simulink model "test_chan_sel"  (Simulink 7.8)
settings: Solver=ode45  StartTime=0.0  StopTime=512  RelTol=1e-3
libraries: xbsIndex_r4 x128, casper_library_misc x14, xps_library x9, simulink x4
settings Model: Creator=dprice  LastModifiedBy=dprice

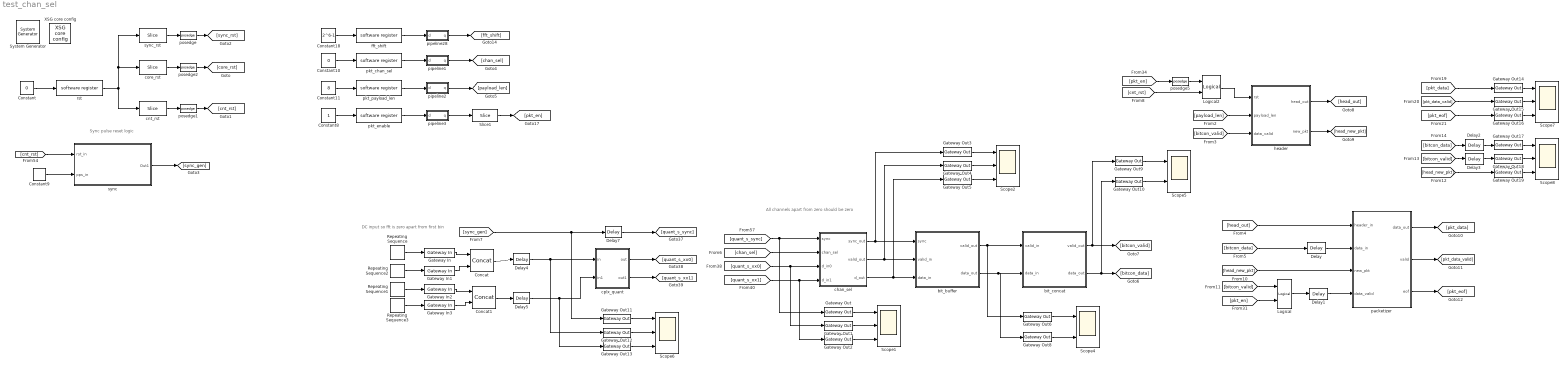
== system test_chan_sel ==
  note: Sync pulse reset logic
  note: DC input so fft is zero apart from first bin
  note: All channels apart from zero should be zero
  " System Generator" : xbsIndex_r4/ System Generator  Tag=genX  xilinxfamily=virtex5  part=xc5vsx95t  speed=-1  package=ff1136  synthesis_tool=XST  clock_wrapper=Clock Enables  directory=./zoom_adc_single_pol/sysgen  proj_type=Project Navigator  Synth_file=XST Defaults  Impl_file=ISE Defaults  testbench=off  simulink_period=1  sysclk_period=5  dcm_input_clock_period=100  incr_netlist=off  trim_vbits=Everywhere in SubSystem  dbl_ovrd=According to Block Masks  core_generation=According to Block Masks  run_coregen=off  deprecated_control=off  eval_field=0  block_type=sysgen
  Concat : xbsIndex_r4/Concat  num_inputs=2  dbl_ovrd=off  block_type=concat
  Concat1 : xbsIndex_r4/Concat  num_inputs=2  dbl_ovrd=off  block_type=concat
  Constant : Constant  Value=0
  Constant10 : Constant  Value=0
  Constant11 : Constant  Value=8
  Constant18 : Constant  Value=2^6-1
  Constant8 : Constant
  Constant9 : xbsIndex_r4/Constant  const=0  gui_display_data_type=Boolean  arith_type=Boolean  n_bits=8  bin_pt=6  preci_type=Single  exp_width=8  frac_width=24  explicit_period=on  period=1  equ=P=C  opselect=C  inp2=PCIN>>17  opr=+  inp1=P  carry=CIN  dbl_ovrd=off  block_type=constant
  Delay{,1..5} (6 alike) : xbsIndex_r4/Delay  rst=off  infoeditControl=Selection of Reset will increase slice count due to use of real FFs and instead of SRLs  en=off  latency=1  dbl_ovrd=off  reg_retiming=off  block_type=delay
  Delay7 : xbsIndex_r4/Delay  rst=off  infoeditControl=Selection of Reset will increase slice count due to use of real FFs and instead of SRLs  en=off  latency=3  dbl_ovrd=off  reg_retiming=off  block_type=delay
  Gateway In{,1..3} (4 alike) : xbsIndex_r4/Gateway In  gui_display_data_type=Fixed-point  arith_type=Unsigned  n_bits=18  bin_pt=0  preci_type=Single  exp_width=8  frac_width=24  quantization="Round  (unbiased: +/- Inf)"  overflow=Saturate  period=1  dbl_ovrd=off  timing_constraint=None  locs_specified=off  LOCs={}  inherit_from_input=off  UseAsADC=off  ADCChannel='1'  hdl_port=on  block_type=gatewayin
      settings: infoedit="Gateway in block.  Converts inputs of type Simulink integer, single, double and fixed point to  Xilinx fixed-point or floating-point data type.<br><br>Hardware notes:  In hardware these blocks become top level input ports."
  Gateway Out{,1..6,8..19} (19 alike) : xbsIndex_r4/Gateway Out  inherit_from_input=off  hdl_port=on  timing_constraint=None  locs_specified=off  LOCs={}  UseAsDAC=off  DACChannel='1'  block_type=gatewayout
      settings: infoedit="Gateway out block.  Converts Xilinx fixed-point or floating-point type inputs into ouputs of type Simulink integer, single, double, or fixed point.<br><br>Hardware notes:  In hardware these blocks become top level output ports or are discarded, depending on how they are configured."
  Logical : xbsIndex_r4/Logical  logical_function=AND  inputs=2  en=off  latency=0  precision=Full  arith_type=Unsigned  n_bits=16  bin_pt=0  align_bp=on  dbl_ovrd=off  block_type=logical
  Logical2 : xbsIndex_r4/Logical  logical_function=OR  inputs=2  en=off  latency=0  precision=Full  arith_type=Unsigned  n_bits=16  bin_pt=0  align_bp=on  dbl_ovrd=off  block_type=logical
  Repeating Sequence : simulink/Sources/Repeating Sequence  rep_seq_t=[1 2 3 4 5 6 7 8 9]  rep_seq_y=[128 0 0 0 0 0 0 0 0]
  Repeating Sequence1 : simulink/Sources/Repeating Sequence  rep_seq_t=[1 2 3 4 5 6 7 8]  rep_seq_y=[0 0 0 0 0 0 0 0]
  Repeating Sequence2 : simulink/Sources/Repeating Sequence  rep_seq_t=[1 2 3 4 5 6 7 8 9]  rep_seq_y=[128 0 0 0 0 0 0 0 0]
  Repeating Sequence3 : simulink/Sources/Repeating Sequence  rep_seq_t=[1 2 3 4 5 6 7 8]  rep_seq_y=[0 0 0 0 0 0 0 0]
  Scope{1..2,6..8} (5 alike) : Scope  NumInputPorts=3
      Scope1 settings: YMin=-5~-5~-5  YMax=5~5~5
      Scope2 settings: YMin=-5~-5~-5  YMax=5~5~5  SaveName=ScopeData6
      Scope6 settings: YMin=-5~-5~-5  YMax=5~5~5  SaveName=ScopeData10
      Scope7 settings: TimeRange=290.1459854014598  YMin=9.44473e+21~0~-1  YMax=3.5e+38~1~1  SaveName=ScopeData11
      Scope8 settings: TimeRange=290.1459854014598  YMin=0~0~0  YMax=1.2e+18~1~1  SaveName=ScopeData12
  Scope4 : Scope  NumInputPorts=2
      settings: YMin=-5~-5  YMax=5~5  SaveName=ScopeData8
  Scope5 : Scope  NumInputPorts=2
      settings: YMin=-5~-5  YMax=5~5  SaveName=ScopeData9
  Slice1 : xbsIndex_r4/Slice  nbits=1  boolean_output=on  mode=Lower Bit Location + Width  bit1=1  base1=MSB of Input  bit0=0  base0=LSB of Input  dbl_ovrd=off  block_type=slice
      settings: block_version=10.1.3
  XSG core config : xps_library/XSG core config  Tag=xps:xsg  hw_sys=ROACH:sx95t  ibob_linux=off  clk_src=adc0_clk  iBOB_clk_src=sys_clk  BEE2_ctrl_clk_src=sys_clk  BEE2_usr_clk_src=sys_clk  ROACH_clk_src=adc0_clk  ROACH2_clk_src=adc0_clk  CORR_clk_src=sys_clk  gpio_clk_io_group=iBOB:sma  gpio_clk_bit_index=0  clk_rate=200  sample_period=1  synthesis_tool=XST  mpc_type=powerpc440_ext
  bit_buffer : Subsystem
  bit_concat : Subsystem
  chan_sel : Subsystem
  cnt_rst : xbsIndex_r4/Slice  nbits=1  boolean_output=on  mode=Lower Bit Location + Width  bit1=0  base1=MSB of Input  bit0=0  base0=LSB of Input  dbl_ovrd=off  block_type=slice
  core_rst : xbsIndex_r4/Slice  nbits=1  boolean_output=on  mode=Lower Bit Location + Width  bit1=0  base1=MSB of Input  bit0=1  base0=LSB of Input  dbl_ovrd=off  block_type=slice
  cplx_quant : Subsystem  AncestorBlock=hipsr_library/quant
  fft_shift : xps_library/software register  Tag=xps:sw_reg  io_dir=From Processor  arith_type=Unsigned  bitwidth=32  bin_pt=0  sample_period=1  gw_name=test_chan_sel_fft_shift_user_data_out
      link override coarse_r01_acc_len_user_data_out: arith_type=Unsigned  n_bits=32  bin_pt=0  period=1
      link override coarse_r02_acc_len_user_data_out: arith_type=Unsigned  n_bits=32  bin_pt=0  period=1
      link override coarse_r03_acc_len_user_data_out: arith_type=Unsigned  n_bits=32  bin_pt=0  period=1
      link override coarse_r04_acc_len_user_data_out: arith_type=Unsigned  n_bits=32  bin_pt=0  period=1
      link override coarse_r06_acc_len_user_data_out: arith_type=Unsigned  n_bits=32  bin_pt=0  period=1
      link override coarse_r07_acc_len_user_data_out: arith_type=Unsigned  n_bits=32  bin_pt=0  period=1
      link override coarse_r08_acc_len_user_data_out: arith_type=Unsigned  n_bits=32  bin_pt=0  period=1
      link override coarse_r09_acc_len_user_data_out: arith_type=Unsigned  n_bits=32  bin_pt=0  period=1
      link override coarse_r10_acc_len_user_data_out: arith_type=Unsigned  n_bits=32  bin_pt=0  period=1
      link override coarse_r12_acc_len_user_data_out: arith_type=Unsigned  n_bits=32  bin_pt=0  period=1
      link override convert: arith_type=Unsigned  n_bits=32  bin_pt=0
      link override qdr_single_r01_acc_len_coarse_user_data_out: arith_type=Unsigned  n_bits=32  bin_pt=0  period=1
      link override qdr_single_r02_acc_len_coarse_user_data_out: arith_type=Unsigned  n_bits=32  bin_pt=0  period=1
      link override qdr_single_r04_acc_len_coarse_user_data_out: arith_type=Unsigned  n_bits=32  bin_pt=0  period=1
      link override r_spec_2048_r102_acc_len_user_data_out: arith_type=Unsigned  n_bits=32  bin_pt=0  period=1
      link override r_spec_2048_r102_nosim_acc_len_user_data_out: arith_type=Unsigned  n_bits=32  bin_pt=0  period=1
      link override r_spec_2048_r103_acc_len_user_data_out: arith_type=Unsigned  n_bits=32  bin_pt=0  period=1
      link override r_spec_2048_r104_acc_len_user_data_out: arith_type=Unsigned  n_bits=32  bin_pt=0  period=1
      link override r_spec_2048_r104_test0_acc_len_user_data_out: arith_type=Unsigned  n_bits=32  bin_pt=0  period=1
      link override r_spec_2048_r104_test_acc_len_user_data_out: arith_type=Unsigned  n_bits=32  bin_pt=0  period=1
      link override r_spec_2048_r105_acc_len_user_data_out: arith_type=Unsigned  n_bits=32  bin_pt=0  period=1
      link override r_spec_test0_acc_len_user_data_out: arith_type=Unsigned  n_bits=32  bin_pt=0  period=1
      link override r_spec_test4_acc_len_user_data_out: arith_type=Unsigned  n_bits=32  bin_pt=0  period=1
      link override roach_spec_acc_len_user_data_out: arith_type=Unsigned  n_bits=32  bin_pt=0  period=1
      link override roach_spec_no10gbe_acc_len_user_data_out: arith_type=Unsigned  n_bits=32  bin_pt=0  period=1
      link override roach_spec_rst_sync_cnt_user_data_out: arith_type=Unsigned  n_bits=32  bin_pt=0  period=1
      link override toast_256ch_16bit_r02_acc_len_user_data_out: arith_type=Unsigned  n_bits=32  bin_pt=0  period=1
      link override toast_256ch_16bit_r04_acc_len_user_data_out: arith_type=Unsigned  n_bits=32  bin_pt=0  period=1
      link override toast_256ch_16bit_r05_acc_len_user_data_out: arith_type=Unsigned  n_bits=32  bin_pt=0  period=1
  header : Subsystem
  packetizer : Subsystem
  pipeline1 : Subsystem  AncestorBlock=casper_library_delays/pipeline  mask(pipeline){latency=1}
      mask help:
      | An explicitly laid-out delay line to avoid mapping to SRL16s
      | for use in pipelining to help achieve timing closure.
      mask init:
      | pipeline_init(gcb,'latency',latency);
      settings: AttributesFormatString=Latency = %<latency>
      mask Display:
      | port_label('input', 1, 'd');
      | port_label('output', 1, 'q');
      | disp(['Z^-', num2str(latency)]);
  pipeline2 : Subsystem  AncestorBlock=casper_library_delays/pipeline  mask(pipeline){latency=1}
      mask help:
      | An explicitly laid-out delay line to avoid mapping to SRL16s
      | for use in pipelining to help achieve timing closure.
      mask init:
      | pipeline_init(gcb,'latency',latency);
      settings: AttributesFormatString=Latency = %<latency>
      mask Display:
      | port_label('input', 1, 'd');
      | port_label('output', 1, 'q');
      | disp(['Z^-', num2str(latency)]);
  pipeline28 : Subsystem  AncestorBlock=casper_library_delays/pipeline  mask(pipeline){latency=1}
      mask help:
      | An explicitly laid-out delay line to avoid mapping to SRL16s
      | for use in pipelining to help achieve timing closure.
      mask init:
      | pipeline_init(gcb,'latency',latency);
      settings: AttributesFormatString=Latency = %<latency>
      mask Display:
      | port_label('input', 1, 'd');
      | port_label('output', 1, 'q');
      | disp(['Z^-', num2str(latency)]);
  pipeline3 : Subsystem  AncestorBlock=casper_library_delays/pipeline  mask(pipeline){latency=1}
      mask help:
      | An explicitly laid-out delay line to avoid mapping to SRL16s
      | for use in pipelining to help achieve timing closure.
      mask init:
      | pipeline_init(gcb,'latency',latency);
      settings: AttributesFormatString=Latency = %<latency>
      mask Display:
      | port_label('input', 1, 'd');
      | port_label('output', 1, 'q');
      | disp(['Z^-', num2str(latency)]);
  pkt_chan_sel : xps_library/software register  Tag=xps:sw_reg  io_dir=From Processor  arith_type=Unsigned  bitwidth=32  bin_pt=0  sample_period=1  gw_name=test_chan_sel_pkt_chan_sel_user_data_out
      link override hipsr_tgbe3_pkt_chan_sel_user_data_out: arith_type=Unsigned  n_bits=32  bin_pt=0  period=1
  pkt_enable : xps_library/software register  Tag=xps:sw_reg  io_dir=From Processor  arith_type=Unsigned  bitwidth=32  bin_pt=0  sample_period=1  gw_name=test_chan_sel_pkt_enable_user_data_out
      link override hipsr_tgbe3_pkt_enable_user_data_out: arith_type=Unsigned  n_bits=32  bin_pt=0  period=1
  pkt_payload_len : xps_library/software register  Tag=xps:sw_reg  io_dir=From Processor  arith_type=Unsigned  bitwidth=32  bin_pt=0  sample_period=1  gw_name=test_chan_sel_pkt_payload_len_user_data_out
      link override hipsr_tgbe3_pkt_payload_len_user_data_out: arith_type=Unsigned  n_bits=32  bin_pt=0  period=1
  posedge{,1..2,5} (4 alike) : casper_library_misc/posedge  Tag=Rising Edge Detector
  rst : xps_library/software register  Tag=xps:sw_reg  io_dir=From Processor  arith_type=Unsigned  bitwidth=32  bin_pt=0  sample_period=1  gw_name=test_chan_sel_rst_user_data_out
      link override hipsr_tgbe3_rst_user_data_out: arith_type=Unsigned  n_bits=32  bin_pt=0  period=1
  sync : Subsystem  AncestorBlock=hipsr_library/sync
  sync_rst : xbsIndex_r4/Slice  nbits=1  boolean_output=on  mode=Lower Bit Location + Width  bit1=0  base1=MSB of Input  bit0=2  base0=LSB of Input  dbl_ovrd=off  block_type=slice
  wires:
  Constant/1 -> rst/1
  rst/1 -> cnt_rst/1, core_rst/1, sync_rst/1
  core_rst/1 -> posedge2/1
  cnt_rst/1 -> posedge1/1
  sync_rst/1 -> posedge/1
  posedge/1 -> [sync_rst]
  posedge1/1 -> [cnt_rst]
  posedge2/1 -> [core_rst]
  Constant9/1 -> sync/2(pps_in)
  sync/1(Out1) -> [sync_gen]
  [cnt_rst] -> sync/1(rst_in)
  Delay7/1 -> [quant_s_sync]
  cplx_quant/1(out) -> [quant_s_xx0]
  cplx_quant/2(out1) -> [quant_s_xx1]
  bit_buffer/2(data_out) -> bit_concat/2(data_in), Gateway Out8/1
  bit_concat/2(data_out) -> [bitcon_data], Gateway Out10/1
  bit_concat/1(valid_out) -> [bitcon_valid], Gateway Out9/1
  [chan_sel] -> chan_sel/2(chan_sel)
  chan_sel/1(sync_out) -> bit_buffer/1(sync), Gateway Out3/1
  chan_sel/2(valid_out) -> bit_buffer/2(valid_in), Gateway Out4/1
  chan_sel/3(d_out) -> bit_buffer/3(data_in), Gateway Out5/1
  bit_buffer/1(valid_out) -> bit_concat/1(valid_in), Gateway Out6/1
  [quant_s_xx0] -> chan_sel/3(d_in0), Gateway Out1/1
  [quant_s_xx1] -> chan_sel/4(d_in1), Gateway Out2/1
  [quant_s_sync] -> chan_sel/1(sync), Gateway Out/1
  Gateway Out/1 -> Scope1/1
  Gateway Out1/1 -> Scope1/2
  Gateway Out2/1 -> Scope1/3
  Gateway Out3/1 -> Scope2/1
  Gateway Out4/1 -> Scope2/2
  Gateway Out5/1 -> Scope2/3
  Gateway Out6/1 -> Scope4/1
  Gateway Out8/1 -> Scope4/2
  Gateway Out9/1 -> Scope5/1
  Gateway Out10/1 -> Scope5/2
  Gateway Out11/1 -> Scope6/1
  Gateway Out12/1 -> Scope6/2
  Gateway Out13/1 -> Scope6/3
  [payload_len] -> header/2(payload_len)
  [bitcon_valid] -> header/3(data_valid)
  header/1(head_out) -> [head_out]
  header/2(new_pkt) -> [head_new_pkt]
  [pkt_en] -> posedge5/1
  posedge5/1 -> Logical2/1
  [cnt_rst] -> Logical2/2
  Logical2/1 -> header/1(rst)
  [head_out] -> packetizer/1(header_in)
  [bitcon_data] -> Delay/1
  [head_new_pkt] -> packetizer/3(new_pkt)
  packetizer/1(data_out) -> [pkt_data]
  packetizer/2(valid) -> [pkt_data_valid]
  packetizer/3(eof) -> [pkt_eof]
  Delay/1 -> packetizer/2(data_in)
  Delay1/1 -> packetizer/4(data_valid)
  [pkt_en] -> Logical/2
  [bitcon_valid] -> Logical/1
  Logical/1 -> Delay1/1
  Gateway Out17/1 -> Scope8/1
  Gateway Out18/1 -> Scope8/2
  Gateway Out19/1 -> Scope8/3
  [bitcon_data] -> Delay2/1
  [bitcon_valid] -> Delay3/1
  [head_new_pkt] -> Gateway Out19/1
  Gateway Out14/1 -> Scope7/1
  Gateway Out15/1 -> Scope7/2
  Gateway Out16/1 -> Scope7/3
  [pkt_data] -> Gateway Out14/1
  [pkt_data_valid] -> Gateway Out15/1
  [pkt_eof] -> Gateway Out16/1
  Delay2/1 -> Gateway Out17/1
  Delay3/1 -> Gateway Out18/1
  Constant10/1 -> pkt_chan_sel/1
  pkt_chan_sel/1 -> pipeline1/1(d)
  Constant11/1 -> pkt_payload_len/1
  pkt_payload_len/1 -> pipeline2/1(d)
  Constant18/1 -> fft_shift/1
  fft_shift/1 -> pipeline28/1(d)
  pipeline28/1(q) -> [fft_shift]
  pipeline1/1(q) -> [chan_sel]
  pipeline2/1(q) -> [payload_len]
  Constant8/1 -> pkt_enable/1
  pkt_enable/1 -> pipeline3/1(d)
  pipeline3/1(q) -> Slice1/1
  Slice1/1 -> [pkt_en]
  Repeating Sequence/1 -> Gateway In/1
  Repeating Sequence1/1 -> Gateway In2/1
  [sync_gen] -> Delay7/1, Gateway Out11/1
  Repeating Sequence2/1 -> Gateway In1/1
  Repeating Sequence3/1 -> Gateway In3/1
  Gateway In/1 -> Concat/1
  Gateway In1/1 -> Concat/2
  Gateway In2/1 -> Concat1/1
  Gateway In3/1 -> Concat1/2
  Concat1/1 -> Delay5/1
  Concat/1 -> Delay4/1
  Delay4/1 -> cplx_quant/1(in), Gateway Out12/1
  Delay5/1 -> cplx_quant/2(in1), Gateway Out13/1

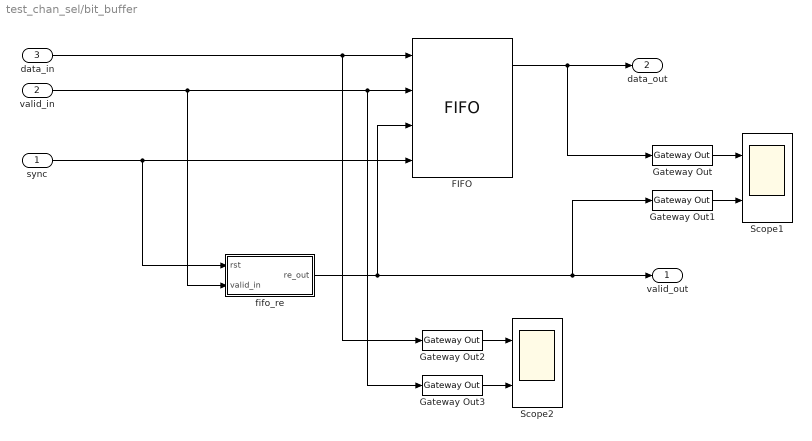
== system test_chan_sel/bit_buffer ==
  sync : Inport
  valid_in : Inport  Port=2
  data_in : Inport  Port=3
  FIFO : xbsIndex_r4/FIFO  performance_options=Standard_FIFO  depth=16  percent_nbits=1  rst=on  en=off  use_dcount=off  use_percent_full_port=off  use_almost_empty=off  almost_empty_thresh=2  use_almost_full=off  almost_full_thresh=14  dbl_ovrd=off  mem_type=Block RAM  explicit_period=off  block_type=fifo
  Gateway Out{,1..3} (4 alike) : xbsIndex_r4/Gateway Out  inherit_from_input=off  hdl_port=on  timing_constraint=None  locs_specified=off  LOCs={}  UseAsDAC=off  DACChannel='1'  block_type=gatewayout
      settings: infoedit="Gateway out block.  Converts Xilinx fixed-point or floating-point type inputs into ouputs of type Simulink integer, single, double, or fixed point.<br><br>Hardware notes:  In hardware these blocks become top level output ports or are discarded, depending on how they are configured."
  Scope1 : Scope  NumInputPorts=2
      settings: YMin=-5~-5  YMax=5~5  SaveName=ScopeData3
  Scope2 : Scope  NumInputPorts=2
      settings: YMin=-5~-5  YMax=5~5  SaveName=ScopeData2
  fifo_re : Subsystem  mask{buf_len=2}
      mask prompts: buf_len "Buffer length (2^N)"
      mask help:
      | Read enabler block for FIFO buffer. Counts for desired number of valid datum,
      | then spits out data in a chunk.
  valid_out : Outport
  data_out : Outport  Port=2
  wires:
  data_in/1 -> FIFO/1, Gateway Out2/1
  valid_in/1 -> fifo_re/2(valid_in), FIFO/2, Gateway Out3/1
  sync/1 -> FIFO/4, fifo_re/1(rst)
  FIFO/1 -> data_out/1, Gateway Out/1
  fifo_re/1(re_out) -> FIFO/3, valid_out/1, Gateway Out1/1
  Gateway Out/1 -> Scope1/1
  Gateway Out1/1 -> Scope1/2
  Gateway Out2/1 -> Scope2/1
  Gateway Out3/1 -> Scope2/2

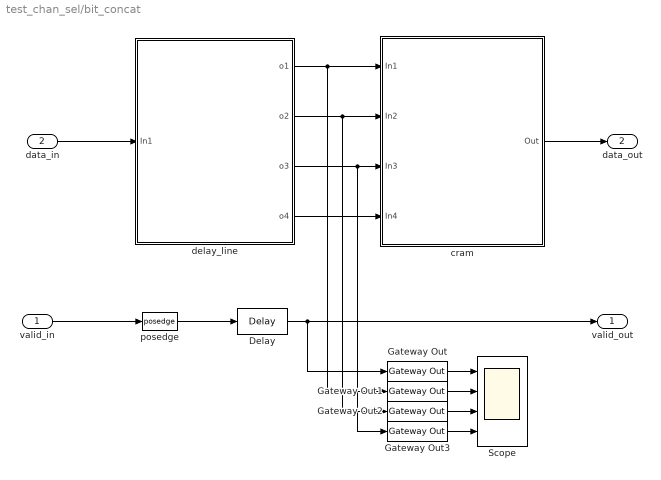
== system test_chan_sel/bit_concat ==
  valid_in : Inport
  data_in : Inport  Port=2
  Delay : xbsIndex_r4/Delay  rst=off  infoeditControl=Selection of Reset will increase slice count due to use of real FFs and instead of SRLs  en=off  latency=7  dbl_ovrd=off  reg_retiming=off  block_type=delay
  Gateway Out{,1..3} (4 alike) : xbsIndex_r4/Gateway Out  inherit_from_input=off  hdl_port=on  timing_constraint=None  locs_specified=off  LOCs={}  UseAsDAC=off  DACChannel='1'  block_type=gatewayout
      settings: infoedit="Gateway out block.  Converts Xilinx fixed-point or floating-point type inputs into ouputs of type Simulink integer, single, double, or fixed point.<br><br>Hardware notes:  In hardware these blocks become top level output ports or are discarded, depending on how they are configured."
  Scope : Scope  NumInputPorts=4
      settings: YMin=-5~-5~-5~-5  YMax=5~5~5~5  SaveName=ScopeData7
  cram : Subsystem  AncestorBlock=gavrt_library/cram  mask(cram){num_slice=4}
      mask prompts: num_slice "Number of slices"
      mask help: Concatenates inputs together after forcing binary point to zero.
      mask init:
      | cram_init(gcb, ...
      |     'num_slice', num_slice);
  delay_line : Subsystem
  posedge : casper_library_misc/posedge  Tag=Rising Edge Detector
  valid_out : Outport
  data_out : Outport  Port=2
  wires:
  data_in/1 -> delay_line/1(In1)
  delay_line/1(o1) -> cram/1(In1), Gateway Out1/1
  delay_line/2(o2) -> cram/2(In2), Gateway Out2/1
  delay_line/3(o3) -> cram/3(In3), Gateway Out3/1
  delay_line/4(o4) -> cram/4(In4)
  valid_in/1 -> posedge/1
  posedge/1 -> Delay/1
  Delay/1 -> valid_out/1, Gateway Out/1
  cram/1(Out) -> data_out/1
  Gateway Out/1 -> Scope/1
  Gateway Out1/1 -> Scope/2
  Gateway Out2/1 -> Scope/3
  Gateway Out3/1 -> Scope/4

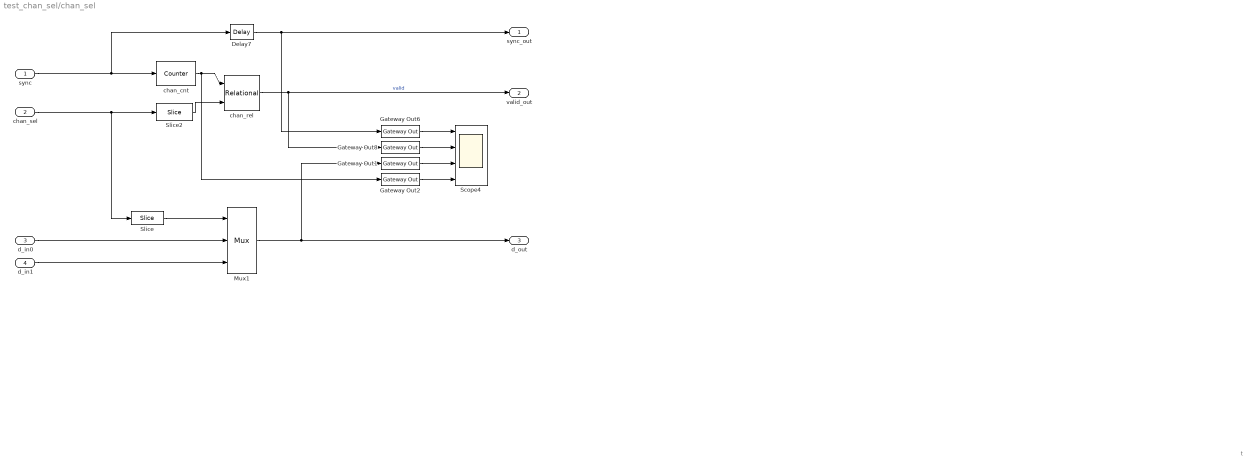
== system test_chan_sel/chan_sel ==
  note: t
  sync : Inport
  chan_sel : Inport  Port=2
  d_in0 : Inport  Port=3
  d_in1 : Inport  Port=4
  Delay7 : xbsIndex_r4/Delay  rst=off  infoeditControl=Selection of Reset will increase slice count due to use of real FFs and instead of SRLs  en=off  latency=1  dbl_ovrd=off  reg_retiming=off  block_type=delay
  Gateway Out{1..2,6,8} (4 alike) : xbsIndex_r4/Gateway Out  inherit_from_input=off  hdl_port=on  timing_constraint=None  locs_specified=off  LOCs={}  UseAsDAC=off  DACChannel='1'  block_type=gatewayout
      settings: infoedit="Gateway out block.  Converts Xilinx fixed-point or floating-point type inputs into ouputs of type Simulink integer, single, double, or fixed point.<br><br>Hardware notes:  In hardware these blocks become top level output ports or are discarded, depending on how they are configured."
  Mux1 : xbsIndex_r4/Mux  inputs=2  en=off  latency=1  precision=Full  arith_type=Unsigned  n_bits=16  bin_pt=14  quantization=Truncate  overflow=Wrap  dbl_ovrd=off  block_type=mux
  Scope4 : Scope  NumInputPorts=4
      settings: YMin=-5~-5~-5~-5  YMax=5~5~5~5  SaveName=ScopeData13
  Slice : xbsIndex_r4/Slice  nbits=1  boolean_output=off  mode=Lower Bit Location + Width  bit1=0  base1=MSB of Input  bit0=0  base0=LSB of Input  dbl_ovrd=off  block_type=slice
  Slice2 : xbsIndex_r4/Slice  nbits=4  boolean_output=off  mode=Lower Bit Location + Width  bit1=1  base1=MSB of Input  bit0=1  base0=LSB of Input  dbl_ovrd=off  block_type=slice
      settings: block_version=10.1.3
  chan_cnt : xbsIndex_r4/Counter  cnt_type=Free Running  cnt_to=Inf  operation=Up  start_count=0  cnt_by_val=1  arith_type=Unsigned  n_bits=3  bin_pt=0  load_pin=off  rst=on  en=off  explicit_period=on  period=1  dbl_ovrd=off  use_behavioral_HDL=off  implementation=Fabric  block_type=counter
  chan_rel : xbsIndex_r4/Relational  mode=a=b  en=off  latency=0  dbl_ovrd=off  block_type=relational
  sync_out : Outport
  valid_out : Outport  Port=2
  d_out : Outport  Port=3
  wires:
  sync/1 -> chan_cnt/1, Delay7/1
  chan_cnt/1 -> chan_rel/1, Gateway Out2/1
  Slice2/1 -> chan_rel/2
  chan_rel/1 -> valid_out/1, Gateway Out8/1  "valid"
  chan_sel/1 -> Slice2/1, Slice/1
  d_in0/1 -> Mux1/2
  d_in1/1 -> Mux1/3
  Mux1/1 -> d_out/1, Gateway Out1/1
  Slice/1 -> Mux1/1
  Gateway Out6/1 -> Scope4/1
  Gateway Out8/1 -> Scope4/2
  Gateway Out1/1 -> Scope4/3
  Gateway Out2/1 -> Scope4/4
  Delay7/1 -> sync_out/1, Gateway Out6/1

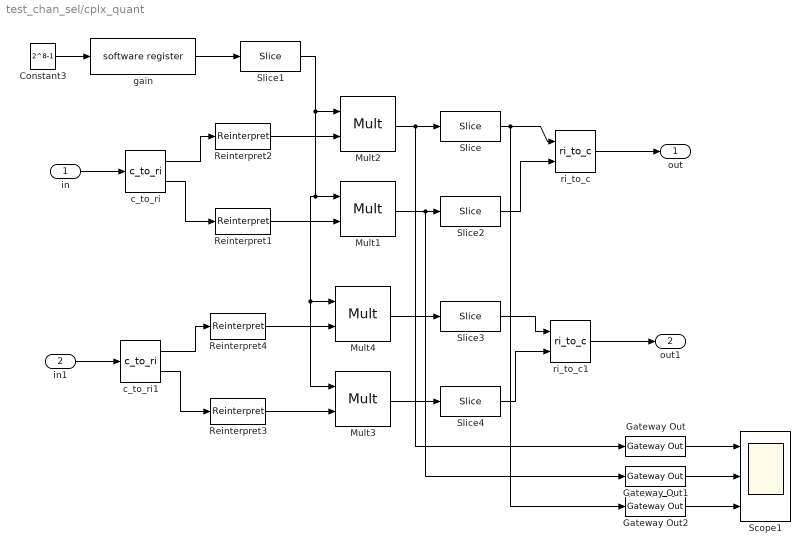
== system test_chan_sel/cplx_quant ==
  in : Inport
  in1 : Inport  Port=2
  Constant3 : Constant  Value=2^8-1
  Gateway Out : xbsIndex_r4/Gateway Out  inherit_from_input=off  hdl_port=on  timing_constraint=None  locs_specified=off  LOCs={}  UseAsDAC=off  DACChannel='1'  block_type=gatewayout
      settings: infoedit="Gateway out block.  Converts Xilinx fixed-point or floating-point type inputs into ouputs of type Simulink integer, single, double, or fixed point.<br><br>Hardware notes:  In hardware these blocks become top level output ports or are discarded, depending on how they are configured."
  Gateway Out1 : xbsIndex_r4/Gateway Out  inherit_from_input=off  hdl_port=on  timing_constraint=None  locs_specified=off  LOCs={}  UseAsDAC=off  DACChannel='1'  block_type=gatewayout
      settings: infoedit="Gateway out block.  Converts Xilinx fixed-point or floating-point type inputs into ouputs of type Simulink integer, single, double, or fixed point.<br><br>Hardware notes:  In hardware these blocks become top level output ports or are discarded, depending on how they are configured."
  Gateway Out2 : xbsIndex_r4/Gateway Out  inherit_from_input=off  hdl_port=on  timing_constraint=None  locs_specified=off  LOCs={}  UseAsDAC=off  DACChannel='1'  block_type=gatewayout
      settings: infoedit="Gateway out block.  Converts Xilinx fixed-point or floating-point type inputs into ouputs of type Simulink integer, single, double, or fixed point.<br><br>Hardware notes:  In hardware these blocks become top level output ports or are discarded, depending on how they are configured."
  Mult{1..4} (4 alike) : xbsIndex_r4/Mult  precision=Full  arith_type="Signed  (2's comp)"  n_bits=16  bin_pt=14  quantization=Truncate  overflow=Wrap  en=off  latency=3  dbl_ovrd=off  use_behavioral_HDL=off  opt=Speed  use_embedded=on  optimum_pipeline=off  pipeline=on  use_rpm=on  placement_style=Triangular  block_type=mult
  Reinterpret{1..4} (4 alike) : xbsIndex_r4/Reinterpret  force_arith_type=on  arith_type="Signed  (2's comp)"  force_bin_pt=on  bin_pt=17  block_type=reinterpret
  Scope1 : Scope  NumInputPorts=3
      settings: YMin=-5~-5~-5  YMax=5~5~5
  Slice{,2..4} (4 alike) : xbsIndex_r4/Slice  nbits=8  boolean_output=off  mode=Upper Bit Location + Width  bit1=-16  base1=MSB of Input  bit0=0  base0=LSB of Input  dbl_ovrd=off  block_type=slice
  Slice1 : xbsIndex_r4/Slice  nbits=16  boolean_output=off  mode=Lower Bit Location + Width  bit1=0  base1=MSB of Input  bit0=0  base0=LSB of Input  dbl_ovrd=off  block_type=slice
  c_to_ri : casper_library_misc/c_to_ri  n_bits=18  bin_pt=17
  c_to_ri1 : casper_library_misc/c_to_ri  n_bits=18  bin_pt=17
  gain : xps_library/software register  Tag=xps:sw_reg  io_dir=From Processor  arith_type=Unsigned  bitwidth=32  bin_pt=0  sample_period=1  gw_name=test_chan_sel_cplx_quant_gain_user_data_out
  ri_to_c : casper_library_misc/ri_to_c
  ri_to_c1 : casper_library_misc/ri_to_c
  out : Outport
  out1 : Outport  Port=2
  wires:
  in/1 -> c_to_ri/1
  c_to_ri/1 -> Reinterpret2/1
  c_to_ri/2 -> Reinterpret1/1
  Slice/1 -> ri_to_c/1, Gateway Out2/1
  Slice2/1 -> ri_to_c/2
  ri_to_c/1 -> out/1
  Slice1/1 -> Mult2/1, Mult1/1, Mult3/1, Mult4/1
  gain/1 -> Slice1/1
  Constant3/1 -> gain/1
  Mult2/1 -> Gateway Out/1, Slice/1
  Reinterpret2/1 -> Mult2/2
  Reinterpret1/1 -> Mult1/2
  Mult1/1 -> Gateway Out1/1, Slice2/1
  in1/1 -> c_to_ri1/1
  c_to_ri1/1 -> Reinterpret4/1
  c_to_ri1/2 -> Reinterpret3/1
  Slice3/1 -> ri_to_c1/1
  Slice4/1 -> ri_to_c1/2
  ri_to_c1/1 -> out1/1
  Mult4/1 -> Slice3/1
  Reinterpret4/1 -> Mult4/2
  Reinterpret3/1 -> Mult3/2
  Mult3/1 -> Slice4/1
  Gateway Out/1 -> Scope1/1
  Gateway Out1/1 -> Scope1/2
  Gateway Out2/1 -> Scope1/3

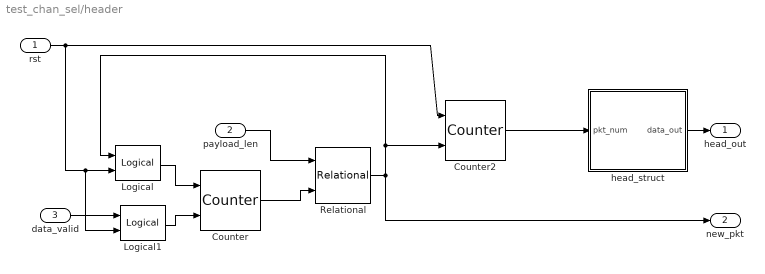
== system test_chan_sel/header ==
  rst : Inport
  payload_len : Inport  Port=2
  data_valid : Inport  Port=3
  Counter : xbsIndex_r4/Counter  cnt_type=Free Running  cnt_to=Inf  operation=Up  start_count=0  cnt_by_val=1  arith_type=Unsigned  n_bits=16  bin_pt=0  load_pin=off  rst=on  en=on  explicit_period=on  period=1  dbl_ovrd=off  use_behavioral_HDL=off  implementation=Fabric  block_type=counter
  Counter2 : xbsIndex_r4/Counter  cnt_type=Free Running  cnt_to=Inf  operation=Up  start_count=0  cnt_by_val=1  arith_type=Unsigned  n_bits=32  bin_pt=0  load_pin=off  rst=on  en=on  explicit_period=on  period=1  dbl_ovrd=off  use_behavioral_HDL=off  implementation=Fabric  block_type=counter
  Logical : xbsIndex_r4/Logical  logical_function=OR  inputs=2  en=off  latency=0  precision=Full  arith_type=Unsigned  n_bits=16  bin_pt=0  align_bp=on  dbl_ovrd=off  block_type=logical
  Logical1 : xbsIndex_r4/Logical  logical_function=OR  inputs=2  en=off  latency=0  precision=Full  arith_type=Unsigned  n_bits=16  bin_pt=0  align_bp=on  dbl_ovrd=off  block_type=logical
  Relational : xbsIndex_r4/Relational  mode=a=b  en=off  latency=0  dbl_ovrd=off  block_type=relational
  head_struct : Subsystem
  head_out : Outport
  new_pkt : Outport  Port=2
  wires:
  Counter/1 -> Relational/2
  Relational/1 -> new_pkt/1, Counter2/2, Logical/1
  Counter2/1 -> head_struct/1(pkt_num)
  head_struct/1(data_out) -> head_out/1
  payload_len/1 -> Relational/1
  rst/1 -> Counter2/1, Logical/2, Logical1/2
  Logical/1 -> Counter/1
  data_valid/1 -> Logical1/1
  Logical1/1 -> Counter/2

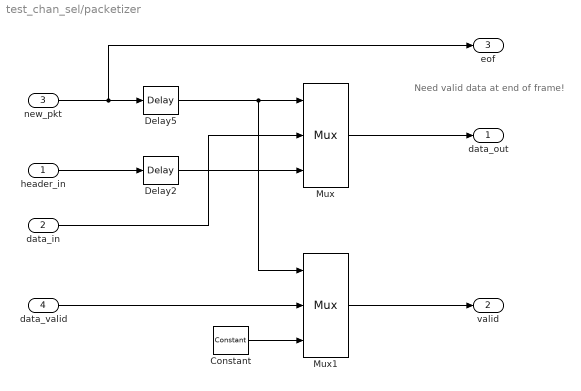
== system test_chan_sel/packetizer ==
  note: Need valid data at end of frame!
  header_in : Inport
  data_in : Inport  Port=2
  new_pkt : Inport  Port=3
  data_valid : Inport  Port=4
  Constant : xbsIndex_r4/Constant  const=1  gui_display_data_type=Boolean  arith_type=Boolean  n_bits=16  bin_pt=14  preci_type=Single  exp_width=8  frac_width=24  explicit_period=on  period=1  equ=P=C  opselect=C  inp2=PCIN>>17  opr=+  inp1=P  carry=CIN  dbl_ovrd=off  block_type=constant
  Delay2 : xbsIndex_r4/Delay  rst=off  infoeditControl=Selection of Reset will increase slice count due to use of real FFs and instead of SRLs  en=off  latency=2  dbl_ovrd=off  reg_retiming=off  block_type=delay
  Delay5 : xbsIndex_r4/Delay  rst=off  infoeditControl=Selection of Reset will increase slice count due to use of real FFs and instead of SRLs  en=off  latency=2  dbl_ovrd=off  reg_retiming=off  block_type=delay
  Mux : xbsIndex_r4/Mux  inputs=2  en=off  latency=0  precision=Full  arith_type=Unsigned  n_bits=16  bin_pt=14  quantization=Truncate  overflow=Wrap  dbl_ovrd=off  block_type=mux
  Mux1 : xbsIndex_r4/Mux  inputs=2  en=off  latency=0  precision=Full  arith_type=Unsigned  n_bits=16  bin_pt=14  quantization=Truncate  overflow=Wrap  dbl_ovrd=off  block_type=mux
  data_out : Outport
  valid : Outport  Port=2
  eof : Outport  Port=3
  wires:
  new_pkt/1 -> Delay5/1, eof/1
  header_in/1 -> Delay2/1
  data_in/1 -> Mux/2
  data_valid/1 -> Mux1/2
  Constant/1 -> Mux1/3
  Mux1/1 -> valid/1
  Mux/1 -> data_out/1
  Delay2/1 -> Mux/3
  Delay5/1 -> Mux/1, Mux1/1

== system test_chan_sel/pipeline1 ==
  d : Inport
  Register0 : xbsIndex_r4/Register  init=0  rst=off  en=off  dbl_ovrd=off  block_type=register
      settings: block_version=11.4
  q : Outport
  wires:
  d/1 -> Register0/1
  Register0/1 -> q/1

== system test_chan_sel/pipeline2 ==
  d : Inport
  Register0 : xbsIndex_r4/Register  init=0  rst=off  en=off  dbl_ovrd=off  block_type=register
      settings: block_version=11.4
  q : Outport
  wires:
  d/1 -> Register0/1
  Register0/1 -> q/1

== system test_chan_sel/pipeline28 ==
  d : Inport
  Register0 : xbsIndex_r4/Register  init=0  rst=off  en=off  dbl_ovrd=off  block_type=register
      settings: block_version=11.4
  q : Outport
  wires:
  d/1 -> Register0/1
  Register0/1 -> q/1

== system test_chan_sel/pipeline3 ==
  d : Inport
  Register0 : xbsIndex_r4/Register  init=0  rst=off  en=off  dbl_ovrd=off  block_type=register
      settings: block_version=11.4
  q : Outport
  wires:
  d/1 -> Register0/1
  Register0/1 -> q/1

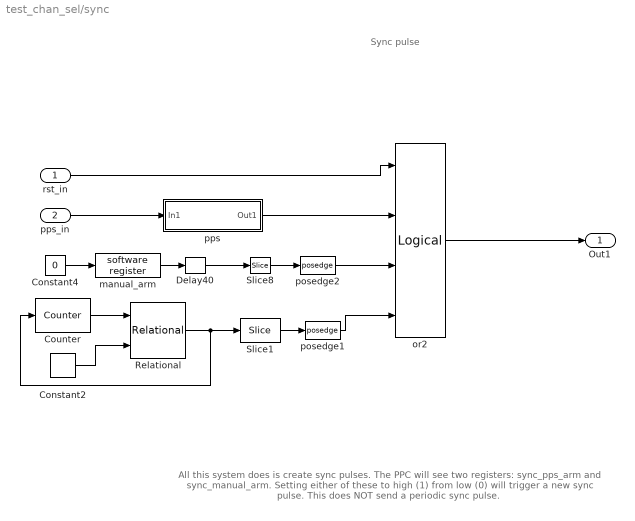
== system test_chan_sel/sync ==
  note: Sync pulse
  note: All this system does is create sync pulses. The PPC will see two registers:
      | sync_pps_arm and sync_manual_arm.
      |
      | Setting either of these to high (1) from low (0) will trigger a new sync pulse.
      | This does NOT send a periodic sync pulse.
  rst_in : Inport
  pps_in : Inport  Port=2
  Constant2 : xbsIndex_r4/Constant  const=1  gui_display_data_type=Fixed-point  arith_type=Signed (2's comp)  n_bits=2  bin_pt=0  preci_type=Single  exp_width=8  frac_width=24  explicit_period=on  period=1  equ=P=C  opselect=C  inp2=PCIN>>17  opr=+  inp1=P  carry=CIN  dbl_ovrd=off  block_type=constant
  Constant4 : Constant  Value=0
  Counter : xbsIndex_r4/Counter  cnt_type=Count Limited  cnt_to=1  operation=Up  start_count=0  cnt_by_val=1  arith_type=Unsigned  n_bits=2  bin_pt=0  load_pin=off  rst=off  en=on  explicit_period=on  period=1  dbl_ovrd=off  use_behavioral_HDL=off  implementation=Fabric  block_type=counter
  Delay40 : xbsIndex_r4/Delay  rst=off  infoeditControl=Selection of Reset will increase slice count due to use of real FFs and instead of SRLs  en=off  latency=1  dbl_ovrd=off  reg_retiming=off  block_type=delay
  Relational : xbsIndex_r4/Relational  mode=a<b  en=off  latency=0  dbl_ovrd=off  block_type=relational
  Slice1 : xbsIndex_r4/Slice  nbits=1  boolean_output=on  mode=Lower Bit Location + Width  bit1=0  base1=MSB of Input  bit0=0  base0=LSB of Input  dbl_ovrd=off  block_type=slice
      settings: block_version=10.1.3
  Slice8 : xbsIndex_r4/Slice  nbits=1  boolean_output=on  mode=Lower Bit Location + Width  bit1=0  base1=MSB of Input  bit0=0  base0=LSB of Input  dbl_ovrd=off  block_type=slice
      settings: block_version=10.1.3
  manual_arm : xps_library/software register  Tag=xps:sw_reg  io_dir=From Processor  arith_type=Unsigned  bitwidth=32  bin_pt=0  sample_period=1  gw_name=test_chan_sel_sync_manual_arm_user_data_out
      link override amnesiac_r100_sync_rst_user_data_out: arith_type=Unsigned  n_bits=32  bin_pt=0  period=1
      link override amnesiac_r101_sync_rst_user_data_out: arith_type=Unsigned  n_bits=32  bin_pt=0  period=1
      link override coarse_r01_sync_rst_user_data_out: arith_type=Unsigned  n_bits=32  bin_pt=0  period=1
      link override coarse_r02_sync_rst_user_data_out: arith_type=Unsigned  n_bits=32  bin_pt=0  period=1
      link override coarse_r03_sync_rst_user_data_out: arith_type=Unsigned  n_bits=32  bin_pt=0  period=1
      link override coarse_r04_sync_rst_user_data_out: arith_type=Unsigned  n_bits=32  bin_pt=0  period=1
      link override coarse_r06_sync_rst_user_data_out: arith_type=Unsigned  n_bits=32  bin_pt=0  period=1
      link override coarse_r07_sync_rst_user_data_out: arith_type=Unsigned  n_bits=32  bin_pt=0  period=1
      link override coarse_r08_sync_rst_user_data_out: arith_type=Unsigned  n_bits=32  bin_pt=0  period=1
      link override coarse_r09_sync_rst_user_data_out: arith_type=Unsigned  n_bits=32  bin_pt=0  period=1
      link override coarse_r10_sync_rst_user_data_out: arith_type=Unsigned  n_bits=32  bin_pt=0  period=1
      link override coarse_r12_sync_rst_user_data_out: arith_type=Unsigned  n_bits=32  bin_pt=0  period=1
      link override convert: arith_type=Unsigned  n_bits=32  bin_pt=0
      link override dpad_spec_r101_acc_len_user_data_out: arith_type=Unsigned  n_bits=32  bin_pt=0  period=1
      link override dpad_spec_r102_acc_len_user_data_out: arith_type=Unsigned  n_bits=32  bin_pt=0  period=1
      link override dpad_spec_r103_acc_len_user_data_out: arith_type=Unsigned  n_bits=32  bin_pt=0  period=1
      link override dpad_spec_r104_acc_len_user_data_out: arith_type=Unsigned  n_bits=32  bin_pt=0  period=1
      link override dpad_spec_r105_acc_len_user_data_out: arith_type=Unsigned  n_bits=32  bin_pt=0  period=1
      link override dpad_spec_r106_fft_shift_user_data_out: arith_type=Unsigned  n_bits=32  bin_pt=0  period=1
      link override dpad_spec_r107_fft_shift_user_data_out: arith_type=Unsigned  n_bits=32  bin_pt=0  period=1
      link override dpad_spec_r108_fft_shift_user_data_out: arith_type=Unsigned  n_bits=32  bin_pt=0  period=1
      link override dpad_spec_r109_fft_shift_user_data_out: arith_type=Unsigned  n_bits=32  bin_pt=0  period=1
      link override dpad_spec_r111_fft_shift_user_data_out: arith_type=Unsigned  n_bits=32  bin_pt=0  period=1
      link override qdr_single_r01_sync_rst_user_data_out: arith_type=Unsigned  n_bits=32  bin_pt=0  period=1
      link override qdr_single_r02_sync_rst_user_data_out: arith_type=Unsigned  n_bits=32  bin_pt=0  period=1
      link override qdr_single_r04_sync_rst_user_data_out: arith_type=Unsigned  n_bits=32  bin_pt=0  period=1
      link override r_spec_2048_r102_acc_len_user_data_out: arith_type=Unsigned  n_bits=32  bin_pt=0  period=1
      link override r_spec_2048_r102_nosim_acc_len_user_data_out: arith_type=Unsigned  n_bits=32  bin_pt=0  period=1
      link override r_spec_2048_r103_acc_len_user_data_out: arith_type=Unsigned  n_bits=32  bin_pt=0  period=1
      link override r_spec_2048_r104_acc_len_user_data_out: arith_type=Unsigned  n_bits=32  bin_pt=0  period=1
      link override r_spec_2048_r104_test0_acc_len_user_data_out: arith_type=Unsigned  n_bits=32  bin_pt=0  period=1
      link override r_spec_2048_r104_test_acc_len_user_data_out: arith_type=Unsigned  n_bits=32  bin_pt=0  period=1
      link override r_spec_2048_r105_acc_len_user_data_out: arith_type=Unsigned  n_bits=32  bin_pt=0  period=1
      link override r_spec_test0_acc_len_user_data_out: arith_type=Unsigned  n_bits=32  bin_pt=0  period=1
      link override r_spec_test4_acc_len_user_data_out: arith_type=Unsigned  n_bits=32  bin_pt=0  period=1
      link override roach_spec_acc_len_user_data_out: arith_type=Unsigned  n_bits=32  bin_pt=0  period=1
      link override roach_spec_no10gbe_acc_len_user_data_out: arith_type=Unsigned  n_bits=32  bin_pt=0  period=1
      link override roach_spec_rst_sync_cnt_user_data_out: arith_type=Unsigned  n_bits=32  bin_pt=0  period=1
      link override the_drowned_world_r100_fft_shift_user_data_out: arith_type=Unsigned  n_bits=32  bin_pt=0  period=1
      link override the_drowned_world_r101_fft_shift_user_data_out: arith_type=Unsigned  n_bits=32  bin_pt=0  period=1
      link override the_drowned_world_r102_fft_shift_user_data_out: arith_type=Unsigned  n_bits=32  bin_pt=0  period=1
      link override the_drowned_world_r103_fft_shift_user_data_out: arith_type=Unsigned  n_bits=32  bin_pt=0  period=1
      link override the_drowned_world_r104_fft_shift_user_data_out: arith_type=Unsigned  n_bits=32  bin_pt=0  period=1
      link override the_drowned_world_r105_sync_rst_user_data_out: arith_type=Unsigned  n_bits=32  bin_pt=0  period=1
      link override the_drowned_world_r106_sync_rst_user_data_out: arith_type=Unsigned  n_bits=32  bin_pt=0  period=1
      link override the_drowned_world_r107_sync_rst_user_data_out: arith_type=Unsigned  n_bits=32  bin_pt=0  period=1
      link override the_drowned_world_r108_sync_rst_user_data_out: arith_type=Unsigned  n_bits=32  bin_pt=0  period=1
      link override the_drowned_world_r109_sync_rst_user_data_out: arith_type=Unsigned  n_bits=32  bin_pt=0  period=1
      link override the_drowned_world_r110_sync_rst_user_data_out: arith_type=Unsigned  n_bits=32  bin_pt=0  period=1
      link override toast_256ch_16bit_r02_sync_rst_user_data_out: arith_type=Unsigned  n_bits=32  bin_pt=0  period=1
      link override toast_256ch_16bit_r04_sync_rst_user_data_out: arith_type=Unsigned  n_bits=32  bin_pt=0  period=1
      link override toast_256ch_16bit_r05_sync_rst_user_data_out: arith_type=Unsigned  n_bits=32  bin_pt=0  period=1
  or2 : xbsIndex_r4/Logical  logical_function=OR  inputs=4  en=off  latency=1  precision=Full  arith_type=Unsigned  n_bits=16  bin_pt=0  align_bp=off  dbl_ovrd=off  block_type=logical
  posedge1 : casper_library_misc/posedge  Tag=Rising Edge Detector
  posedge2 : casper_library_misc/posedge  Tag=Rising Edge Detector
  pps : Subsystem
  Out1 : Outport
  wires:
  manual_arm/1 -> Delay40/1
  Delay40/1 -> Slice8/1
  Slice8/1 -> posedge2/1
  pps/1(Out1) -> or2/2
  posedge2/1 -> or2/3
  rst_in/1 -> or2/1
  or2/1 -> Out1/1
  pps_in/1 -> pps/1(In1)
  Constant4/1 -> manual_arm/1
  Slice1/1 -> posedge1/1
  posedge1/1 -> or2/4
  Counter/1 -> Relational/1
  Relational/1 -> Slice1/1, Counter/1
  Constant2/1 -> Relational/2

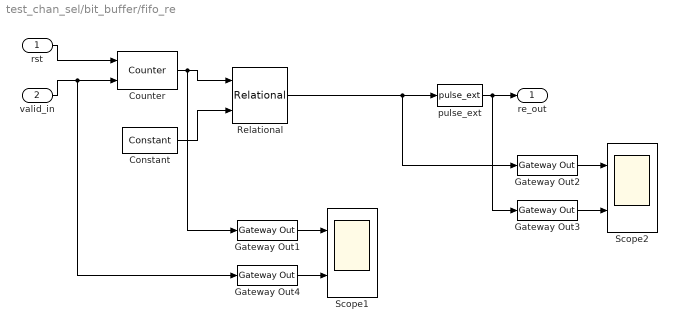
== system test_chan_sel/bit_buffer/fifo_re ==
  rst : Inport
  valid_in : Inport  Port=2
  Constant : xbsIndex_r4/Constant  const=2^(buf_len)-1  gui_display_data_type=Fixed-point  arith_type=Unsigned  n_bits=buf_len+1  bin_pt=0  preci_type=Single  exp_width=8  frac_width=24  explicit_period=on  period=1  equ=P=C  opselect=C  inp2=PCIN>>17  opr=+  inp1=P  carry=CIN  dbl_ovrd=off  block_type=constant
  Counter : xbsIndex_r4/Counter  cnt_type=Free Running  cnt_to=Inf  operation=Up  start_count=0  cnt_by_val=1  arith_type=Unsigned  n_bits=buf_len  bin_pt=0  load_pin=off  rst=on  en=on  explicit_period=on  period=1  dbl_ovrd=off  use_behavioral_HDL=off  implementation=Fabric  block_type=counter
  Gateway Out{1..4} (4 alike) : xbsIndex_r4/Gateway Out  inherit_from_input=off  hdl_port=on  timing_constraint=None  locs_specified=off  LOCs={}  UseAsDAC=off  DACChannel='1'  block_type=gatewayout
      settings: infoedit="Gateway out block.  Converts Xilinx fixed-point or floating-point type inputs into ouputs of type Simulink integer, single, double, or fixed point.<br><br>Hardware notes:  In hardware these blocks become top level output ports or are discarded, depending on how they are configured."
  Relational : xbsIndex_r4/Relational  mode=a=b  en=off  latency=0  dbl_ovrd=off  block_type=relational
  Scope1 : Scope  NumInputPorts=2
      settings: YMin=-5~-5  YMax=5~5  SaveName=ScopeData5
  Scope2 : Scope  NumInputPorts=2
      settings: TimeRange=24.5585874799358  YMin=0~0  YMax=1~1  SaveName=ScopeData4
  pulse_ext : casper_library_misc/pulse_ext  pulse_len=2^(buf_len)
  re_out : Outport
  wires:
  Counter/1 -> Relational/1, Gateway Out1/1
  Constant/1 -> Relational/2
  rst/1 -> Counter/1
  valid_in/1 -> Counter/2, Gateway Out4/1
  Relational/1 -> pulse_ext/1, Gateway Out2/1
  pulse_ext/1 -> re_out/1, Gateway Out3/1
  Gateway Out2/1 -> Scope2/1
  Gateway Out3/1 -> Scope2/2
  Gateway Out1/1 -> Scope1/1
  Gateway Out4/1 -> Scope1/2

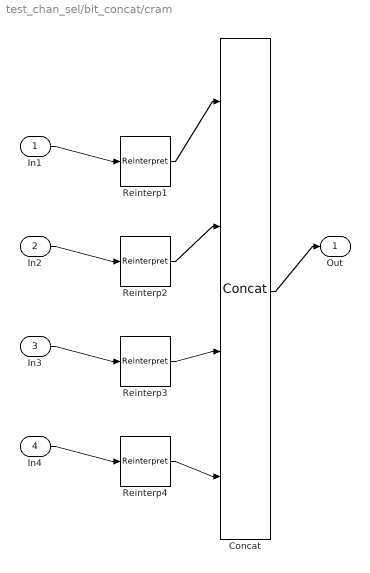
== system test_chan_sel/bit_concat/cram ==
  In1 : Inport
  In2 : Inport  Port=2
  In3 : Inport  Port=3
  In4 : Inport  Port=4
  Concat : xbsIndex_r4/Concat  num_inputs=4  dbl_ovrd=off  block_type=concat
      settings: block_version=10.1.2
  Reinterp{1..4} (4 alike) : xbsIndex_r4/Reinterpret  force_arith_type=on  arith_type=Unsigned  force_bin_pt=on  bin_pt=0  block_type=reinterpret
      settings: infoedit="Changes signal type without altering the binary representation.   You can changed the signal between signed and unsigned, and relocate the binary point.<P><P>Hardware notes: In hardware this block costs nothing.<P><P>Example:  Suppose the input is 6 bits wide, signed, with 2 fractional bits, and the output is forced to unsigned with 0 fractional bits.  Then an input of -2.0 (1110.00 in binary 2's complement) becomes an output of 56 (111000 in binary)."  block_version=10.1.2
  Out : Outport
  wires:
  Concat/1 -> Out/1
  In1/1 -> Reinterp1/1
  Reinterp1/1 -> Concat/1
  In2/1 -> Reinterp2/1
  Reinterp2/1 -> Concat/2
  In3/1 -> Reinterp3/1
  Reinterp3/1 -> Concat/3
  In4/1 -> Reinterp4/1
  Reinterp4/1 -> Concat/4

== system test_chan_sel/bit_concat/delay_line ==
  In1 : Inport
  Delay4 : xbsIndex_r4/Delay  rst=off  infoeditControl=Selection of Reset will increase slice count due to use of real FFs and instead of SRLs  en=off  latency=1  dbl_ovrd=off  reg_retiming=off  block_type=delay
  Delay5 : xbsIndex_r4/Delay  rst=off  infoeditControl=Selection of Reset will increase slice count due to use of real FFs and instead of SRLs  en=off  latency=1  dbl_ovrd=off  reg_retiming=off  block_type=delay
  Delay7 : xbsIndex_r4/Delay  rst=off  infoeditControl=Selection of Reset will increase slice count due to use of real FFs and instead of SRLs  en=off  latency=1  dbl_ovrd=off  reg_retiming=off  block_type=delay
  o1 : Outport
  o2 : Outport  Port=2
  o3 : Outport  Port=3
  o4 : Outport  Port=4
  wires:
  In1/1 -> Delay4/1, o4/1
  Delay4/1 -> Delay5/1, o3/1
  Delay5/1 -> Delay7/1, o2/1
  Delay7/1 -> o1/1

== system test_chan_sel/header/head_struct ==
  pkt_num : Inport
  beam_id : xbsIndex_r4/Constant  const=1  gui_display_data_type=Fixed-point  arith_type=Unsigned  n_bits=8  bin_pt=0  preci_type=Single  exp_width=8  frac_width=24  explicit_period=on  period=1  equ=P=C  opselect=C  inp2=PCIN>>17  opr=+  inp1=P  carry=CIN  dbl_ovrd=off  block_type=constant
  cram : Subsystem  AncestorBlock=gavrt_library/cram  mask(cram){num_slice=5}
      mask prompts: num_slice "Number of slices"
      mask help: Concatenates inputs together after forcing binary point to zero.
      mask init:
      | cram_init(gcb, ...
      |     'num_slice', num_slice);
  diode_state : xbsIndex_r4/Constant  const=0  gui_display_data_type=Fixed-point  arith_type=Unsigned  n_bits=8  bin_pt=0  preci_type=Single  exp_width=8  frac_width=24  explicit_period=on  period=1  equ=P=C  opselect=C  inp2=PCIN>>17  opr=+  inp1=P  carry=CIN  dbl_ovrd=off  block_type=constant
  freq_state : xbsIndex_r4/Constant  const=0  gui_display_data_type=Fixed-point  arith_type=Unsigned  n_bits=8  bin_pt=0  preci_type=Single  exp_width=8  frac_width=24  explicit_period=on  period=1  equ=P=C  opselect=C  inp2=PCIN>>17  opr=+  inp1=P  carry=CIN  dbl_ovrd=off  block_type=constant
  version : xbsIndex_r4/Constant  const=1  gui_display_data_type=Fixed-point  arith_type=Unsigned  n_bits=8  bin_pt=0  preci_type=Single  exp_width=8  frac_width=24  explicit_period=on  period=1  equ=P=C  opselect=C  inp2=PCIN>>17  opr=+  inp1=P  carry=CIN  dbl_ovrd=off  block_type=constant
  data_out : Outport
  wires:
  version/1 -> cram/1(In1)
  beam_id/1 -> cram/2(In2)
  diode_state/1 -> cram/4(In4)
  freq_state/1 -> cram/5(In5)
  cram/1(Out) -> data_out/1
  pkt_num/1 -> cram/3(In3)

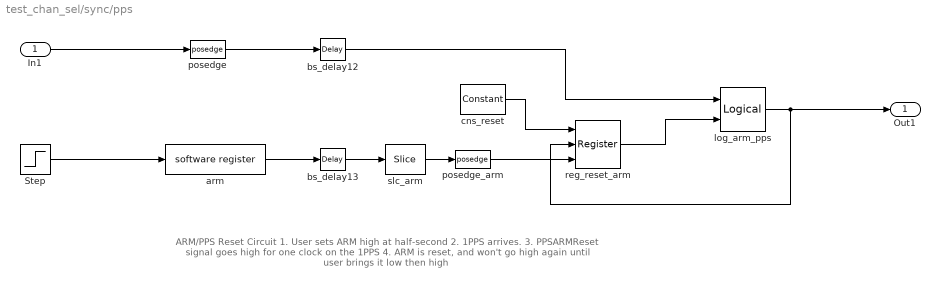
== system test_chan_sel/sync/pps ==
  note: ARM/PPS Reset Circuit
      | 1. User sets ARM high at half-second
      | 2. 1PPS arrives.
      | 3. PPSARMReset signal goes high for one clock on the 1PPS
      | 4. ARM is reset, and won't go high again until user brings it low then high
  In1 : Inport
  Step : Step  SampleTime=0
  arm : xps_library/software register  Tag=xps:sw_reg  io_dir=From Processor  arith_type=Unsigned  bitwidth=32  bin_pt=0  sample_period=1  gw_name=test_chan_sel_sync_pps_arm_user_data_out
      link override adc_to_10gbe_mod_reg_arm_user_data_out: arith_type=Unsigned  n_bits=32  bin_pt=0  period=1
      link override adc_to_10gbe_reg_arm_user_data_out: arith_type=Unsigned  n_bits=32  bin_pt=0  period=1
  bs_delay12 : xbsIndex_r4/Delay  rst=off  infoeditControl=Selection of Reset will increase slice count due to use of real FFs and instead of SRLs  en=off  latency=0  dbl_ovrd=off  reg_retiming=off  block_type=delay
      settings: xl_area=[0, 0, 0, 0, 0, 0, 0]  block_version=10.1
  bs_delay13 : xbsIndex_r4/Delay  rst=off  infoeditControl=Selection of Reset will increase slice count due to use of real FFs and instead of SRLs  en=off  latency=0  dbl_ovrd=off  reg_retiming=off  block_type=delay
      settings: xl_area=[0, 0, 0, 0, 0, 0, 0]  block_version=10.1
  cns_reset : xbsIndex_r4/Constant  const=1  gui_display_data_type=Fixed-point  arith_type=Boolean  n_bits=1  bin_pt=0  preci_type=Single  exp_width=8  frac_width=24  explicit_period=on  period=1  equ=P=C  opselect=C  inp2=PCIN>>17  opr=+  inp1=P  carry=CIN  dbl_ovrd=off  block_type=constant
      settings: block_version=10.1
  log_arm_pps : xbsIndex_r4/Logical  logical_function=AND  inputs=2  en=off  latency=0  precision=Full  arith_type=Unsigned  n_bits=8  bin_pt=2  align_bp=on  dbl_ovrd=off  block_type=logical
      settings: xl_area=[0, 0, 0, 0, 0, 0, 0]  block_version=10.1
  posedge : casper_library_misc/posedge  Tag=Rising Edge Detector
  posedge_arm : casper_library_misc/posedge  Tag=Rising Edge Detector
  reg_reset_arm : xbsIndex_r4/Register  init=0  rst=on  en=on  dbl_ovrd=off  block_type=register
      settings: xl_area=[0, 0, 0, 0, 0, 0, 0]  block_version=10.1
  slc_arm : xbsIndex_r4/Slice  nbits=1  boolean_output=on  mode=Lower Bit Location + Width  bit1=0  base1=MSB of Input  bit0=0  base0=LSB of Input  dbl_ovrd=off  block_type=slice
      settings: infoedit="Extracts a given range of bits from each input sample and presents it at the output.  The output type is ordinarily unsigned with binary point at zero, but can be Boolean when the slice is one bit wide.<P><P>Hardware notes: In hardware this block costs nothing."  block_version=10.1
  Out1 : Outport
  wires:
  arm/1 -> bs_delay13/1
  cns_reset/1 -> reg_reset_arm/1
  reg_reset_arm/1 -> log_arm_pps/2
  log_arm_pps/1 -> reg_reset_arm/2, Out1/1
  slc_arm/1 -> posedge_arm/1
  posedge_arm/1 -> reg_reset_arm/3
  Step/1 -> arm/1
  bs_delay12/1 -> log_arm_pps/1
  bs_delay13/1 -> slc_arm/1
  In1/1 -> posedge/1
  posedge/1 -> bs_delay12/1

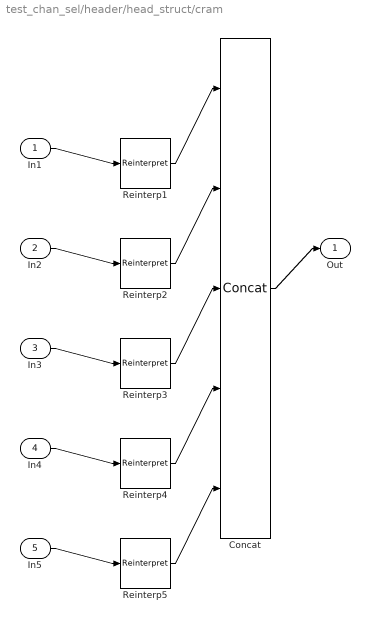
== system test_chan_sel/header/head_struct/cram ==
  In1 : Inport
  In2 : Inport  Port=2
  In3 : Inport  Port=3
  In4 : Inport  Port=4
  In5 : Inport  Port=5
  Concat : xbsIndex_r4/Concat  num_inputs=5  dbl_ovrd=off  block_type=concat
      settings: block_version=10.1.2
  Reinterp{1..5} (5 alike) : xbsIndex_r4/Reinterpret  force_arith_type=on  arith_type=Unsigned  force_bin_pt=on  bin_pt=0  block_type=reinterpret
      Reinterp1 settings: infoedit="Changes signal type without altering the binary representation.   You can changed the signal between signed and unsigned, and relocate the binary point.<P><P>Hardware notes: In hardware this block costs nothing.<P><P>Example:  Suppose the input is 6 bits wide, signed, with 2 fractional bits, and the output is forced to unsigned with 0 fractional bits.  Then an input of -2.0 (1110.00 in binary 2's complement) becomes an output of 56 (111000 in binary)."  block_version=10.1.2
      Reinterp2 settings: infoedit="Changes signal type without altering the binary representation.   You can changed the signal between signed and unsigned, and relocate the binary point.<P><P>Hardware notes: In hardware this block costs nothing.<P><P>Example:  Suppose the input is 6 bits wide, signed, with 2 fractional bits, and the output is forced to unsigned with 0 fractional bits.  Then an input of -2.0 (1110.00 in binary 2's complement) becomes an output of 56 (111000 in binary)."  block_version=10.1.2
      Reinterp3 settings: infoedit="Changes signal type without altering the binary representation.   You can changed the signal between signed and unsigned, and relocate the binary point.<P><P>Hardware notes: In hardware this block costs nothing.<P><P>Example:  Suppose the input is 6 bits wide, signed, with 2 fractional bits, and the output is forced to unsigned with 0 fractional bits.  Then an input of -2.0 (1110.00 in binary 2's complement) becomes an output of 56 (111000 in binary)."  block_version=10.1.2
      Reinterp4 settings: infoedit="Changes signal type without altering the binary representation.   You can changed the signal between signed and unsigned, and relocate the binary point.<P><P>Hardware notes: In hardware this block costs nothing.<P><P>Example:  Suppose the input is 6 bits wide, signed, with 2 fractional bits, and the output is forced to unsigned with 0 fractional bits.  Then an input of -2.0 (1110.00 in binary 2's complement) becomes an output of 56 (111000 in binary)."  block_version=10.1.2
  Out : Outport
  wires:
  Concat/1 -> Out/1
  In1/1 -> Reinterp1/1
  Reinterp1/1 -> Concat/1
  In2/1 -> Reinterp2/1
  Reinterp2/1 -> Concat/2
  In3/1 -> Reinterp3/1
  Reinterp3/1 -> Concat/3
  In4/1 -> Reinterp4/1
  Reinterp4/1 -> Concat/4
  In5/1 -> Reinterp5/1
  Reinterp5/1 -> Concat/5
